simulink model "Connection"  (R2022a)
settings: Solver=VariableStepAuto  StartTime=0.0  StopTime=150  RelTol=1e-3
values from neighbouring files (symbols this model uses):
  scramInit = 93    [Setup.m]
libraries: simulink x10, dspsrcs4 x7, hdlsllib x4, whdlutilities x3, whdledac x3
settings Model: Creator=Zeyan Wu  LastModifiedBy=Zeyan

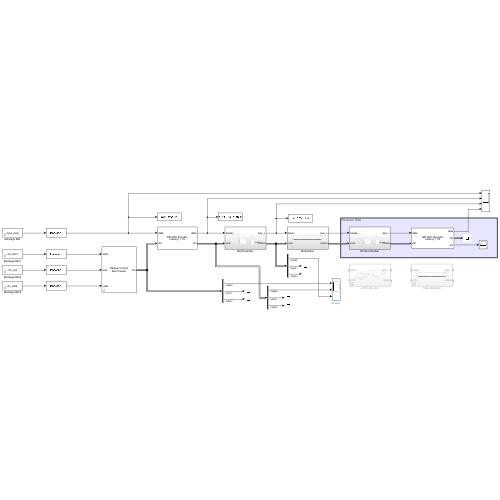
[thumbnail: Simulink's stored preview of the top-level diagram]
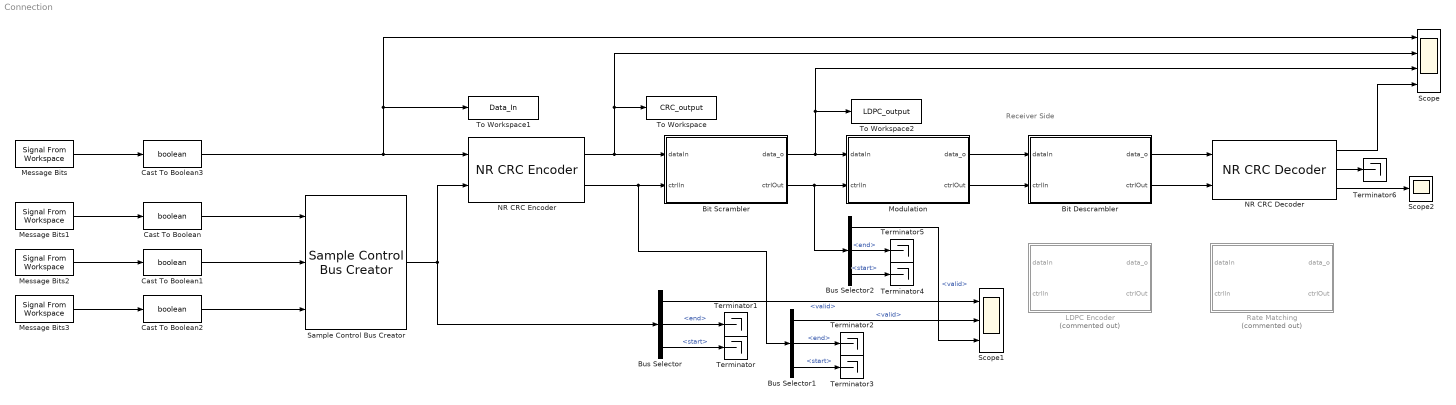
== system Connection ==
  note: Receiver Side
  Bit Descrambler : Subsystem
  Bit Scrambler : Subsystem
  Bus Selector : BusSelector  OutputSignals=valid,end,start
  Bus Selector1 : BusSelector  OutputSignals=valid,end,start
  Bus Selector2 : BusSelector  OutputSignals=valid,end,start
  Cast To Boolean{,1..3} (4 alike) : DataTypeConversion  OutDataTypeStr=boolean  SaturateOnIntegerOverflow=off  RndMeth=Floor
  LDPC Encoder : Subsystem  Commented=on
  Message Bits : dspsrcs4/Signal From Workspace  X=input_msg  Ts=1  nsamps=1  OutputAfterFinalValue=Setting to zero  ignoreOrWarnInputAndFrameLengths=off  OutputFrames=on
  Message Bits1 : dspsrcs4/Signal From Workspace  X=ctrl_start  Ts=1  nsamps=1  OutputAfterFinalValue=Setting to zero  ignoreOrWarnInputAndFrameLengths=off  OutputFrames=on
  Message Bits2 : dspsrcs4/Signal From Workspace  X=ctrl_end  Ts=1  nsamps=1  OutputAfterFinalValue=Setting to zero  ignoreOrWarnInputAndFrameLengths=off  OutputFrames=on
  Message Bits3 : dspsrcs4/Signal From Workspace  X=ctrl_valid  Ts=1  nsamps=1  OutputAfterFinalValue=Setting to zero  ignoreOrWarnInputAndFrameLengths=off  OutputFrames=on
  Modulation : Subsystem
  NR CRC Decoder : whdledac/NR CRC Decoder  CRCType=CRC16  FullCheckSum=off  EnableCRCMaskPort=off  SimulateUsing=Code generation
      settings: SourceProductBaseCode=LH
  NR CRC Encoder : whdledac/NR CRC Encoder  CRCType=CRC16  EnableCRCMaskPort=off  SimulateUsing=Code generation
      settings: SourceProductBaseCode=LH
  Rate Matching : Subsystem  Commented=on
  Sample Control Bus Creator : whdlutilities/Sample Control Bus Creator
      settings: SourceProductBaseCode=LH
  Scope : Scope  NumInputPorts=4
  Scope1 : Scope  NumInputPorts=3
  Scope2 : Scope
  Terminator{,1..6} (7 alike) : Terminator
  To Workspace : ToWorkspace  VariableName=CRC_output  SampleTime=1
      settings: Save2DSignal=2-D array (concatenate along first dimension)
  To Workspace1 : ToWorkspace  VariableName=Data_In  SampleTime=1
      settings: Save2DSignal=2-D array (concatenate along first dimension)
  To Workspace2 : ToWorkspace  VariableName=LDPC_output  SampleTime=1
      settings: Save2DSignal=2-D array (concatenate along first dimension)
  wires:
  Message Bits2/1 -> Cast To Boolean1/1
  Message Bits1/1 -> Cast To Boolean/1
  Message Bits3/1 -> Cast To Boolean2/1
  Sample Control Bus Creator/1 -> Bus Selector/1, NR CRC Encoder/2
  Cast To Boolean/1 -> Sample Control Bus Creator/1
  Cast To Boolean1/1 -> Sample Control Bus Creator/2
  Cast To Boolean2/1 -> Sample Control Bus Creator/3
  Bus Selector/1 -> Scope1/1  "<valid>"
  Bus Selector/3 -> Terminator/1  "<start>"
  NR CRC Encoder/1 -> Bit Scrambler/1(dataIn), Scope/2, To Workspace/1
  Bus Selector/2 -> Terminator1/1  "<end>"
  Message Bits/1 -> Cast To Boolean3/1
  Cast To Boolean3/1 -> Scope/1, To Workspace1/1, NR CRC Encoder/1
  Bus Selector1/2 -> Terminator2/1  "<end>"
  NR CRC Encoder/2 -> Bit Scrambler/2(ctrlIn), Bus Selector1/1
  Bus Selector1/3 -> Terminator3/1  "<start>"
  Bus Selector1/1 -> Scope1/2  "<valid>"
  Bus Selector2/2 -> Terminator5/1  "<end>"
  Bus Selector2/3 -> Terminator4/1  "<start>"
  Bus Selector2/1 -> Scope1/3  "<valid>"
  Bit Scrambler/1(data_o) -> To Workspace2/1, Scope/3, Modulation/1(dataIn)
  Bit Scrambler/2(ctrlOut) -> Modulation/2(ctrlIn), Bus Selector2/1
  Bit Descrambler/1(data_o) -> NR CRC Decoder/1
  Modulation/1(data_o) -> Bit Descrambler/1(dataIn)
  Modulation/2(ctrlOut) -> Bit Descrambler/2(ctrlIn)
  Bit Descrambler/2(ctrlOut) -> NR CRC Decoder/2
  NR CRC Decoder/1 -> Scope/4
  NR CRC Decoder/2 -> Terminator6/1
  NR CRC Decoder/3 -> Scope2/1

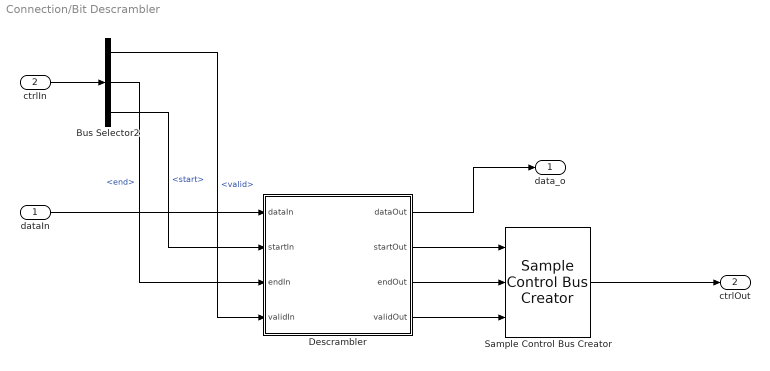
== system Connection/Bit Descrambler ==
  dataIn : Inport
  ctrlIn : Inport  Port=2
  Bus Selector2 : BusSelector  OutputSignals=valid,end,start
  Descrambler : Subsystem
  Sample Control Bus Creator : whdlutilities/Sample Control Bus Creator
      settings: SourceProductBaseCode=LH
  data_o : Outport
  ctrlOut : Outport  Port=2
  wires:
  dataIn/1 -> Descrambler/1(dataIn)
  Descrambler/1(dataOut) -> data_o/1
  ctrlIn/1 -> Bus Selector2/1
  Bus Selector2/1 -> Descrambler/4(validIn)  "<valid>"
  Bus Selector2/2 -> Descrambler/3(endIn)  "<end>"
  Bus Selector2/3 -> Descrambler/2(startIn)  "<start>"
  Descrambler/2(startOut) -> Sample Control Bus Creator/1
  Descrambler/3(endOut) -> Sample Control Bus Creator/2
  Descrambler/4(validOut) -> Sample Control Bus Creator/3
  Sample Control Bus Creator/1 -> ctrlOut/1

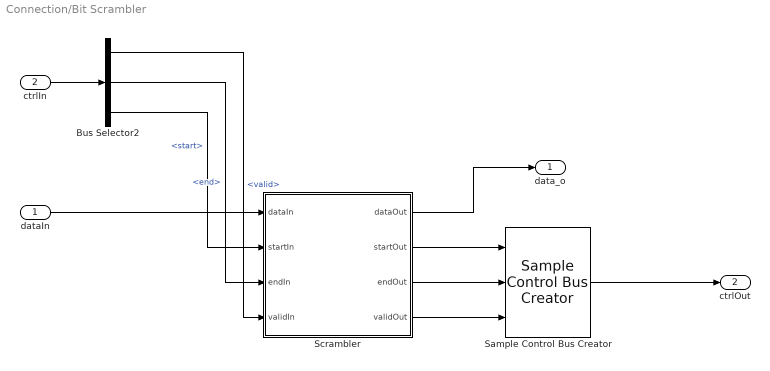
== system Connection/Bit Scrambler ==
  dataIn : Inport
  ctrlIn : Inport  Port=2
  Bus Selector2 : BusSelector  OutputSignals=valid,end,start
  Sample Control Bus Creator : whdlutilities/Sample Control Bus Creator
      settings: SourceProductBaseCode=LH
  Scrambler : Subsystem
  data_o : Outport
  ctrlOut : Outport  Port=2
  wires:
  dataIn/1 -> Scrambler/1(dataIn)
  Scrambler/1(dataOut) -> data_o/1
  ctrlIn/1 -> Bus Selector2/1
  Bus Selector2/1 -> Scrambler/4(validIn)  "<valid>"
  Bus Selector2/2 -> Scrambler/3(endIn)  "<end>"
  Bus Selector2/3 -> Scrambler/2(startIn)  "<start>"
  Scrambler/2(startOut) -> Sample Control Bus Creator/1
  Scrambler/3(endOut) -> Sample Control Bus Creator/2
  Scrambler/4(validOut) -> Sample Control Bus Creator/3
  Sample Control Bus Creator/1 -> ctrlOut/1

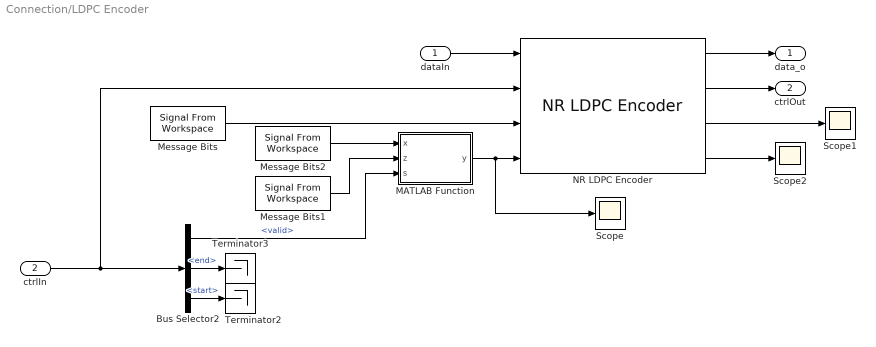
== system Connection/LDPC Encoder ==
  dataIn : Inport
  ctrlIn : Inport  Port=2
  Bus Selector2 : BusSelector  OutputSignals=valid,end,start
  MATLAB Function : MATLAB Function  TreatAsAtomicUnit=on
  Message Bits : dspsrcs4/Signal From Workspace  X=BGN  Ts=1  nsamps=1  OutputAfterFinalValue=Holding final value  ignoreOrWarnInputAndFrameLengths=off  OutputFrames=on
  Message Bits1 : dspsrcs4/Signal From Workspace  X=liftingSize  Ts=1  nsamps=1  OutputAfterFinalValue=Holding final value  ignoreOrWarnInputAndFrameLengths=off  OutputFrames=on
  Message Bits2 : dspsrcs4/Signal From Workspace  X=liftingSize_zero  Ts=1  nsamps=1  OutputAfterFinalValue=Holding final value  ignoreOrWarnInputAndFrameLengths=off  OutputFrames=on
  NR LDPC Encoder : whdledac/NR LDPC Encoder
      settings: SourceProductBaseCode=LH
  Scope : Scope
  Scope1 : Scope
  Scope2 : Scope
  Terminator2 : Terminator
  Terminator3 : Terminator
  data_o : Outport
  ctrlOut : Outport  Port=2
  wires:
  NR LDPC Encoder/2 -> ctrlOut/1
  dataIn/1 -> NR LDPC Encoder/1
  NR LDPC Encoder/1 -> data_o/1
  NR LDPC Encoder/3 -> Scope1/1
  NR LDPC Encoder/4 -> Scope2/1
  Message Bits/1 -> NR LDPC Encoder/3
  ctrlIn/1 -> NR LDPC Encoder/2, Bus Selector2/1
  Bus Selector2/3 -> Terminator2/1  "<start>"
  Bus Selector2/2 -> Terminator3/1  "<end>"
  Bus Selector2/1 -> MATLAB Function/3(s)  "<valid>"
  MATLAB Function/1(y) -> Scope/1, NR LDPC Encoder/4
  Message Bits2/1 -> MATLAB Function/1(x)
  Message Bits1/1 -> MATLAB Function/2(z)

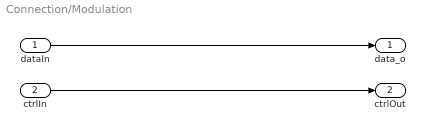
== system Connection/Modulation ==
  dataIn : Inport
  ctrlIn : Inport  Port=2
  data_o : Outport
  ctrlOut : Outport  Port=2
  wires:
  dataIn/1 -> data_o/1
  ctrlIn/1 -> ctrlOut/1

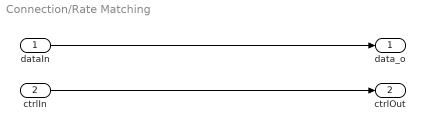
== system Connection/Rate Matching ==
  dataIn : Inport
  ctrlIn : Inport  Port=2
  data_o : Outport
  ctrlOut : Outport  Port=2
  wires:
  dataIn/1 -> data_o/1
  ctrlIn/1 -> ctrlOut/1

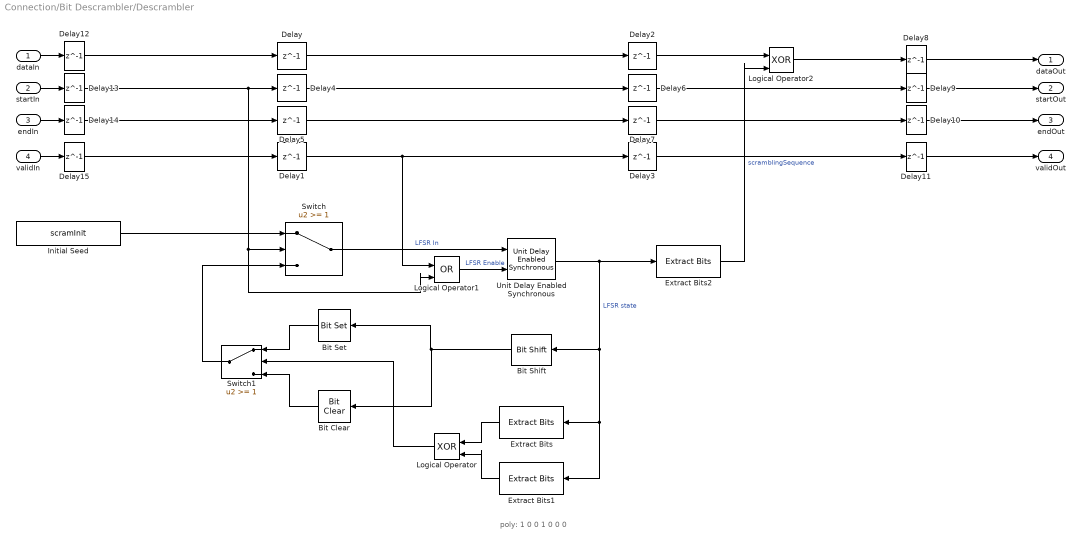
== system Connection/Bit Descrambler/Descrambler ==
  note: poly: 1 0 0 1 0 0 0
  dataIn : Inport
  startIn : Inport  Port=2
  endIn : Inport  Port=3
  validIn : Inport  Port=4
  Bit Clear : simulink/Logic and Bit Operations/Bit Clear  iBit=0
      settings: SourceProductBaseCode=SL
  Bit Set : simulink/Logic and Bit Operations/Bit Set  iBit=0
      settings: SourceProductBaseCode=SL
  Bit Shift : hdlsllib/Logic and Bit Operations/Bit Shift  mode=Shift Left Logical  N=1
  Delay{,1..7} (8 alike) : Delay  DelayLength=1
  Delay{8..15} (8 alike) : Delay  DelayLength=1  InitialCondition=0
  Extract Bits : simulink/Logic and Bit Operations/Extract Bits  bitsToExtract=Range of bits  numBits=8  bitIdxRange=3  outScalingMode=Preserve fixed-point scaling
  Extract Bits1 : simulink/Logic and Bit Operations/Extract Bits  bitsToExtract=Range of bits  numBits=8  bitIdxRange=6  outScalingMode=Preserve fixed-point scaling
  Extract Bits2 : simulink/Logic and Bit Operations/Extract Bits  bitsToExtract=Range of bits  numBits=8  bitIdxRange=0  outScalingMode=Preserve fixed-point scaling
  Initial Seed : Constant  Value=scramInit  OutDataTypeStr=fixdt(0,7,0)  SampleTime=-1
  Logical Operator : Logic  Operator=XOR  IconShape=distinctive  AllPortsSameDT=off  OutDataTypeStr=boolean
  Logical Operator1 : Logic  Operator=OR  IconShape=distinctive  AllPortsSameDT=off  OutDataTypeStr=boolean
  Logical Operator2 : Logic  Operator=XOR  IconShape=distinctive  AllPortsSameDT=off  OutDataTypeStr=boolean
  Switch : Switch  Threshold=1  SaturateOnIntegerOverflow=off  InputSameDT=off
  Switch1 : Switch  Threshold=1  SaturateOnIntegerOverflow=off  InputSameDT=off
  Unit Delay Enabled Synchronous : hdlsllib/Discrete/Unit Delay Enabled Synchronous  InitialCondition=0.0  SampleTime=-1
      settings: SourceProductBaseCode=SL
  dataOut : Outport
  startOut : Outport  Port=2
  endOut : Outport  Port=3
  validOut : Outport  Port=4
  wires:
  Delay15/1 -> Delay1/1
  Delay14/1 -> Delay5/1
  Delay13/1 -> Delay4/1, Switch/2, Logical Operator1/2
  Delay12/1 -> Delay/1
  Delay11/1 -> validOut/1
  Delay10/1 -> endOut/1
  Delay9/1 -> startOut/1
  Delay8/1 -> dataOut/1
  Delay7/1 -> Delay10/1
  Delay6/1 -> Delay9/1
  Delay5/1 -> Delay7/1
  Delay4/1 -> Delay6/1
  endIn/1 -> Delay14/1
  Delay3/1 -> Delay11/1
  Delay2/1 -> Logical Operator2/1
  Logical Operator2/1 -> Delay8/1
  Delay1/1 -> Delay3/1, Logical Operator1/1
  Delay/1 -> Delay2/1
  Logical Operator1/1 -> Unit Delay Enabled Synchronous/2  "LFSR Enable"
  Switch1/1 -> Switch/3
  Bit Shift/1 -> Bit Set/1, Bit Clear/1
  Logical Operator/1 -> Switch1/2
  Bit Clear/1 -> Switch1/3
  Bit Set/1 -> Switch1/1
  Extract Bits1/1 -> Logical Operator/2
  Extract Bits/1 -> Logical Operator/1
  Extract Bits2/1 -> Logical Operator2/2  "scramblingSequence"
  dataIn/1 -> Delay12/1
  Unit Delay Enabled Synchronous/1 -> Extract Bits2/1, Extract Bits/1, Extract Bits1/1, Bit Shift/1  "LFSR state"
  validIn/1 -> Delay15/1
  Initial Seed/1 -> Switch/1
  Switch/1 -> Unit Delay Enabled Synchronous/1  "LFSR In"
  startIn/1 -> Delay13/1

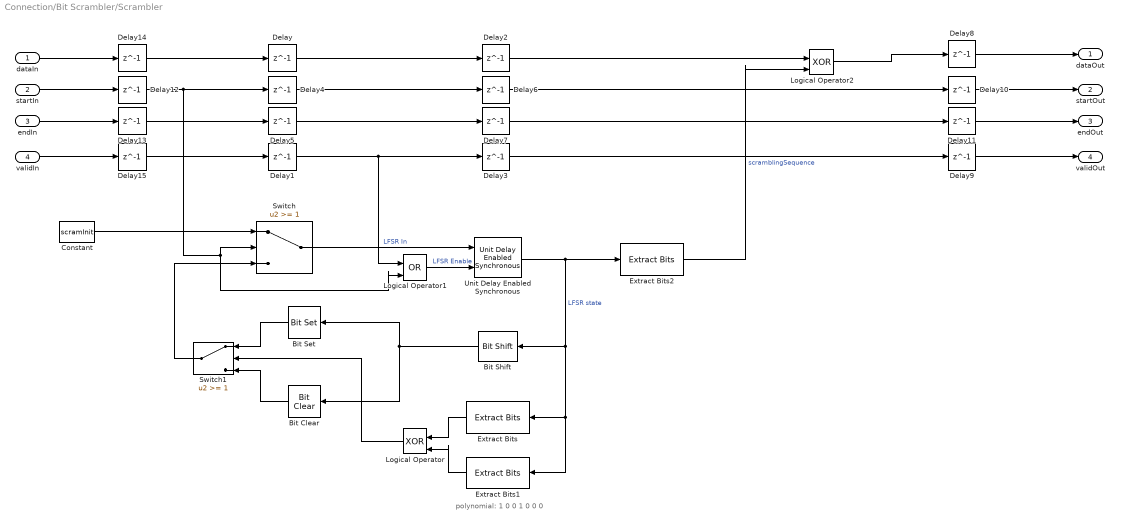
== system Connection/Bit Scrambler/Scrambler ==
  note: polynomial: 1 0 0 1 0 0 0
  dataIn : Inport
  startIn : Inport  Port=2
  endIn : Inport  Port=3
  validIn : Inport  Port=4
  Bit Clear : simulink/Logic and Bit Operations/Bit Clear  iBit=0
      settings: SourceProductBaseCode=SL
  Bit Set : simulink/Logic and Bit Operations/Bit Set  iBit=0
      settings: SourceProductBaseCode=SL
  Bit Shift : hdlsllib/Logic and Bit Operations/Bit Shift  mode=Shift Left Logical  N=1
  Constant : Constant  Value=scramInit  OutDataTypeStr=fixdt(0,7,0)  SampleTime=-1
  Delay{,1..15} (16 alike) : Delay  DelayLength=1
  Extract Bits : simulink/Logic and Bit Operations/Extract Bits  bitsToExtract=Range of bits  numBits=8  bitIdxRange=3  outScalingMode=Preserve fixed-point scaling
  Extract Bits1 : simulink/Logic and Bit Operations/Extract Bits  bitsToExtract=Range of bits  numBits=8  bitIdxRange=6  outScalingMode=Preserve fixed-point scaling
  Extract Bits2 : simulink/Logic and Bit Operations/Extract Bits  bitsToExtract=Range of bits  numBits=8  bitIdxRange=0  outScalingMode=Preserve fixed-point scaling
  Logical Operator : Logic  Operator=XOR  IconShape=distinctive  AllPortsSameDT=off  OutDataTypeStr=boolean
  Logical Operator1 : Logic  Operator=OR  IconShape=distinctive  AllPortsSameDT=off  OutDataTypeStr=boolean
  Logical Operator2 : Logic  Operator=XOR  IconShape=distinctive  AllPortsSameDT=off  OutDataTypeStr=boolean
  Switch : Switch  Threshold=1  SaturateOnIntegerOverflow=off  InputSameDT=off
  Switch1 : Switch  Threshold=1  SaturateOnIntegerOverflow=off  InputSameDT=off
  Unit Delay Enabled Synchronous : hdlsllib/Discrete/Unit Delay Enabled Synchronous  InitialCondition=0.0  SampleTime=-1
      settings: SourceProductBaseCode=SL
  dataOut : Outport
  startOut : Outport  Port=2
  endOut : Outport  Port=3
  validOut : Outport  Port=4
  wires:
  Switch/1 -> Unit Delay Enabled Synchronous/1  "LFSR In"
  Delay13/1 -> Delay5/1
  Delay12/1 -> Delay4/1, Switch/2, Logical Operator1/2
  startIn/1 -> Delay12/1
  Delay15/1 -> Delay1/1
  Extract Bits1/1 -> Logical Operator/2
  Delay14/1 -> Delay/1
  Delay2/1 -> Logical Operator2/1
  Switch1/1 -> Switch/3
  Delay7/1 -> Delay11/1
  Delay/1 -> Delay2/1
  Delay1/1 -> Logical Operator1/1, Delay3/1
  Logical Operator/1 -> Switch1/2
  Bit Clear/1 -> Switch1/3
  Logical Operator1/1 -> Unit Delay Enabled Synchronous/2  "LFSR Enable"
  Bit Set/1 -> Switch1/1
  Delay3/1 -> Delay9/1
  dataIn/1 -> Delay14/1
  validIn/1 -> Delay15/1
  Constant/1 -> Switch/1
  Extract Bits/1 -> Logical Operator/1
  endIn/1 -> Delay13/1
  Unit Delay Enabled Synchronous/1 -> Bit Shift/1, Extract Bits1/1, Extract Bits/1, Extract Bits2/1  "LFSR state"
  Bit Shift/1 -> Bit Clear/1, Bit Set/1
  Delay5/1 -> Delay7/1
  Delay4/1 -> Delay6/1
  Extract Bits2/1 -> Logical Operator2/2  "scramblingSequence"
  Delay6/1 -> Delay10/1
  Logical Operator2/1 -> Delay8/1
  Delay8/1 -> dataOut/1
  Delay10/1 -> startOut/1
  Delay11/1 -> endOut/1
  Delay9/1 -> validOut/1

== matlab function Connection/LDPC Encoder/MATLAB Function ==
  data: x input; y output; z input; s input
function y = selector(x, z, s)
    if(s == false)
        y = x;
    else
        y = z;
    end
end
